simulink model "Controlled_PlanarRobot"  (R2021a)
settings: Solver=ode4  StartTime=0.0  StopTime=10  FixedStep=0.001  MaxStep=0.001  RelTol=1e-3
undefined symbols (not defined in the file): g, I1, I2, kr1, kr2, l1, lc1, lc2, m1, m2, th1, th1p1, th2, th2p1
settings Model: Creator=BODENBURG  LastModifiedBy=aka
settings DebuggingCC: AlgebraicLoopMsg=none  SFMachineParentedDataDiag=warning
settings SFSimCC: CustomCodeUndefinedFunction=UseInterfaceOnly

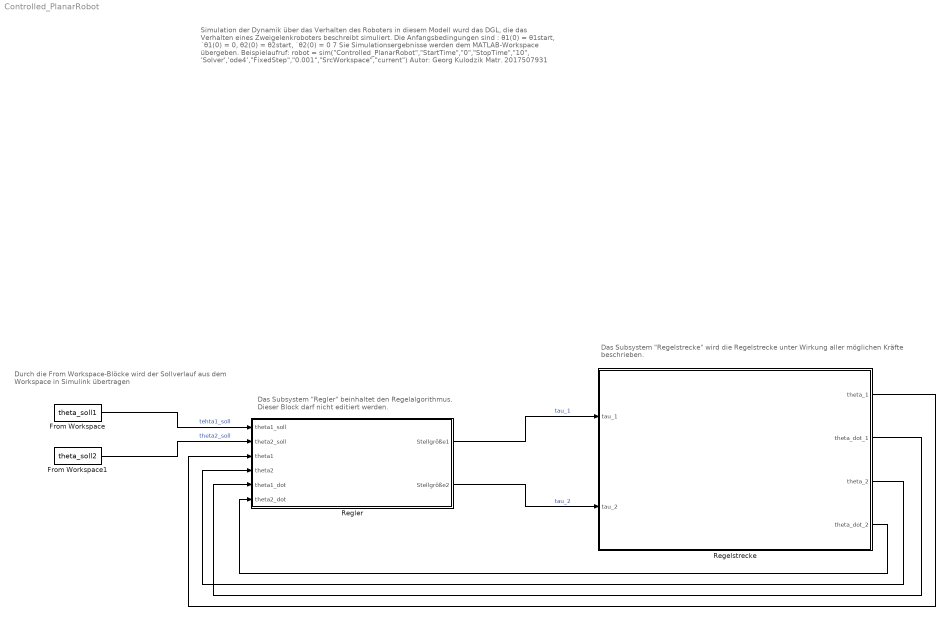
== system Controlled_PlanarRobot ==
  note: Durch die From Workspace-Blöcke wird der Sollverlauf aus dem Workspace in Simulink übertragen
  note: Das Subsystem "Regler" beinhaltet den Regelalgorithmus. Dieser Block darf nicht editiert werden.
  note: Simulation der Dynamik über das Verhalten des Roboters
      | in diesem Modell wurd das DGL,
      |
      | die das Verhalten eines Zweigelenkroboters beschreibt simuliert.
      | Die Anfangsbedingungen sind : θ1(0) = θ1start, ˙θ1(0) = 0, θ2(0) = θ2start, ˙θ2(0) = 0 7
      | Sie Simulationsergebnisse werden dem MATLAB-Workspace übergeben.
      |
      | Beispielaufruf: robot = sim("Controlled_PlanarRobot","StartTime","0","StopTime","10", 'Solver','ode4',"FixedStep","0.001","SrcWorkspace","current")
      |
      | Autor: Georg Kulodzik Matr. 2017507931
  note: Das Subsystem "Regelstrecke" wird die Regelstrecke unter Wirkung aller möglichen Kräfte beschrieben.
  From Workspace : FromWorkspace  VariableName=theta_soll1  OutputAfterFinalValue=Holding final value
  From Workspace1 : FromWorkspace  VariableName=theta_soll2  OutputAfterFinalValue=Holding final value
  Regelstrecke : Subsystem
  Regler : Subsystem
  wires:
  Regelstrecke/1(theta_1) -> Regler/3(theta1)
  Regelstrecke/3(theta_2) -> Regler/4(theta2)
  Regelstrecke/2(theta_dot_1) -> Regler/5(theta1_dot)
  Regelstrecke/4(theta_dot_2) -> Regler/6(theta2_dot)
  Regler/1(Stellgröße1) -> Regelstrecke/1(tau_1)  "tau_1"
  Regler/2(Stellgröße2) -> Regelstrecke/2(tau_2)  "tau_2"
  From Workspace/1 -> Regler/1(theta1_soll)  "tehta1_soll"
  From Workspace1/1 -> Regler/2(theta2_soll)  "theta2_soll"

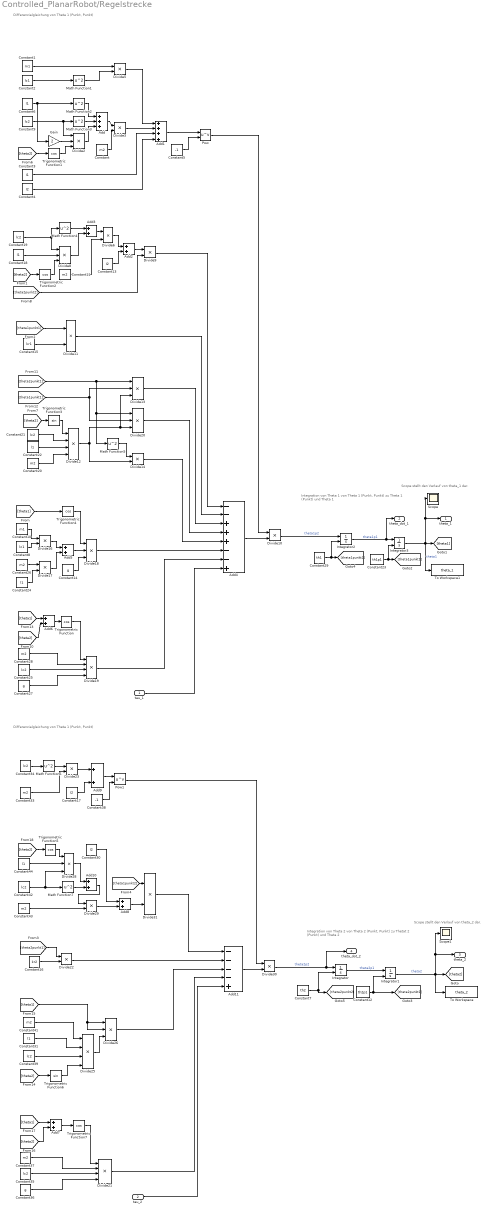
== system Controlled_PlanarRobot/Regelstrecke ==
  note: Integration von Theta 1 von Theta 1 (Punkt, Punkt)
      | zu Theta 1 (Punkt) und Theta 1
  note: Integration von Theta 2 von Theta 2 (Punkt, Punkt)
      | zu Thetat 2 (Punkt) und Theta 2
  note: Scope stellt den Verlauf von theta_1 dar.
  note: Scope stellt den Verlauf von theta_2 dar.
  note: Differenzialgleichung von Theta 1 (Punkt, Punkt)
  note: Differenzialgleichung von Theta 1 (Punkt, Punkt)
  tau_1 : Inport
  tau_2 : Inport  Port=2
  Add : Sum  Inputs=+++
  Add1 : Sum  Inputs=++++
  Add{2..3,5..10} (8 alike) : Sum
  Add11 : Sum  Inputs=----+
  Add4 : Sum  Inputs=--+++--+
  Constant{,11,20,26,28,33,37,41,43} (9 alike) : Constant  Value=m2
  Constant1 : Constant  Value=m1
  Constant10 : Constant  Value=m1
  Constant12 : Constant  Value=th2p1
  Constant{4,13,17,30} (4 alike) : Constant  Value=I2
  Constant14 : Constant  Value=g
  Constant15 : Constant  Value=kr1
  Constant16 : Constant  Value=kr2
  Constant{6,18,22,24,31,44} (6 alike) : Constant  Value=l1
  Constant{9,19,21,25,34..35,39,42} (8 alike) : Constant  Value=lc2
  Constant2 : Constant  Value=lc1
  Constant23 : Constant  Value=th1p1
  Constant27 : Constant  Value=g
  Constant29 : Constant  Value=th1
  Constant3 : Constant  Value=I1
  Constant36 : Constant  Value=g
  Constant38 : Constant  Value=-1
  Constant5 : Constant  Value=-1
  Constant7 : Constant  Value=th2
  Constant8 : Constant  Value=lc1
  Divide{3,5..6,9..11,14,16..17,22..23,29..31} (14 alike) : Product  Inputs=**
  Divide{12,19,21,25} (4 alike) : Product  Inputs=****
  Divide{2,8,13,18,20,26,28} (7 alike) : Product  Inputs=***
  Gain : Gain  Gain=2
  Integrator{,1..3} (4 alike) : Integrator  InitialConditionSource=external
  Math Function{1..7} (7 alike) : Math  Operator=square  SaturateOnIntegerOverflow=on
  Pow : Math  Operator=pow  SignedPower=on  RndMeth=Zero  SaturateOnIntegerOverflow=on
  Pow1 : Math  Operator=pow  SignedPower=on  RndMeth=Zero  SaturateOnIntegerOverflow=on
  Scope : Scope
  Scope1 : Scope
  To Workspace : ToWorkspace  VariableName=theta_2  SaveFormat=Timeseries  SampleTime=-1
  To Workspace1 : ToWorkspace  VariableName=theta_1  SaveFormat=Timeseries  SampleTime=-1
  Trigonometric Function{,1..2,4..5,7} (6 alike) : Trigonometry  Operator=cos
  Trigonometric Function3 : Trigonometry
  Trigonometric Function6 : Trigonometry
  theta_1 : Outport
  theta_dot_1 : Outport  Port=2
  theta_2 : Outport  Port=3
  theta_dot_2 : Outport  Port=4
  wires:
  Constant6/1 -> Math Function2/1, Gain/1
  Constant9/1 -> Math Function3/1, Divide2/1
  Trigonometric Function1/1 -> Divide2/3
  [theta2] -> Trigonometric Function1/1
  Divide2/1 -> Add/3
  Gain/1 -> Divide2/2
  Add/1 -> Divide3/1
  Constant/1 -> Divide3/2
  Constant1/1 -> Divide5/1
  Divide5/1 -> Add1/1
  Divide3/1 -> Add1/2
  Constant3/1 -> Add1/3
  Constant4/1 -> Add1/4
  Add1/1 -> Pow/1
  Constant5/1 -> Pow/2
  Divide6/1 -> Add2/1
  Constant13/1 -> Add2/2
  Constant11/1 -> Divide6/2
  Add3/1 -> Divide6/1
  Constant19/1 -> Math Function4/1, Divide8/1
  Divide8/1 -> Add3/2
  [theta2] -> Trigonometric Function2/1
  Trigonometric Function2/1 -> Divide8/3
  Constant18/1 -> Divide8/2
  [theta2punkt2] -> Divide9/2
  Pow/1 -> Divide10/1
  Add4/1 -> Divide10/2
  Add2/1 -> Divide9/1
  Constant15/1 -> Divide11/2
  [theta1punkt1] -> Divide11/1
  Constant20/1 -> Divide12/4
  Constant22/1 -> Divide12/3
  Constant21/1 -> Divide12/2
  [theta2] -> Trigonometric Function3/1
  Trigonometric Function3/1 -> Divide12/1
  Divide12/1 -> Divide14/2, Divide13/3, Divide20/3
  [theta2punkt1] -> Divide13/1, Math Function5/1, Divide20/1
  Constant10/1 -> Divide16/1
  Constant8/1 -> Divide16/2
  Constant26/1 -> Divide17/1
  Constant24/1 -> Divide17/2
  Divide16/1 -> Add5/1
  Divide17/1 -> Add5/2
  Add5/1 -> Divide18/2
  Trigonometric Function4/1 -> Divide18/1
  [theta1] -> Trigonometric Function4/1
  Constant14/1 -> Divide18/3
  Constant27/1 -> Divide19/4
  Constant25/1 -> Divide19/3
  Constant28/1 -> Divide19/2
  Trigonometric Function/1 -> Divide19/1
  [theta1] -> Add6/1
  [theta2] -> Add6/2
  Add6/1 -> Trigonometric Function/1
  Divide9/1 -> Add4/1
  Divide11/1 -> Add4/2
  Divide13/1 -> Add4/3
  [theta1punkt1] -> Divide13/2, Divide20/2
  Divide20/1 -> Add4/4
  Divide14/1 -> Add4/5
  Divide18/1 -> Add4/6
  tau_1/1 -> Add4/8
  Trigonometric Function7/1 -> Divide21/1
  Constant35/1 -> Divide21/3
  [theta1] -> Add7/1
  Add7/1 -> Trigonometric Function7/1
  Constant37/1 -> Divide21/2
  Constant36/1 -> Divide21/4
  [theta2] -> Add7/2
  Divide19/1 -> Add4/7
  [theta2punkt1] -> Divide22/1
  Constant33/1 -> Divide23/2
  Divide23/1 -> Add9/1
  Constant17/1 -> Add9/2
  Add9/1 -> Pow1/1
  Constant38/1 -> Pow1/2
  Constant41/1 -> Divide25/1
  Constant31/1 -> Divide25/2
  Constant39/1 -> Divide25/3
  [theta2] -> Trigonometric Function6/1
  Trigonometric Function6/1 -> Divide25/4
  Divide25/1 -> Divide26/3
  [theta1] -> Divide26/1, Divide26/2
  Constant16/1 -> Divide22/2
  Constant42/1 -> Divide28/3, Math Function7/1
  Divide28/1 -> Add10/1
  Constant44/1 -> Divide28/2
  Add10/1 -> Divide29/1
  Constant43/1 -> Divide29/2
  Divide22/1 -> Add11/2
  Divide26/1 -> Add11/3
  Divide21/1 -> Add11/4
  tau_2/1 -> Add11/5
  Pow1/1 -> Divide30/1
  Add11/1 -> Divide30/2
  Divide30/1 -> theta_dot_2/1, Integrator/1  "theta2p2"
  Integrator/1 -> Integrator1/1  "theta2p1"
  Constant7/1 -> Integrator/2, [theta2punkt2]
  Constant12/1 -> Integrator1/2, [theta2punkt1]
  Constant23/1 -> Integrator3/2, [theta1punkt1]
  Integrator2/1 -> theta_dot_1/1, Integrator3/1  "theta1p1"
  Constant29/1 -> [theta1punkt2], Integrator2/2
  Divide10/1 -> Integrator2/1  "theta1p2"
  Integrator3/1 -> Scope/1, theta_1/1, To Workspace1/1, [theta1]  "theta1"
  Integrator1/1 -> To Workspace/1, Scope1/1, theta_2/1, [theta2]  "theta2"
  Divide29/1 -> Add8/2
  Constant30/1 -> Add8/1
  Divide31/1 -> Add11/1
  Add8/1 -> Divide31/2
  [theta1punkt2] -> Divide31/1
  [theta2] -> Trigonometric Function5/1
  Trigonometric Function5/1 -> Divide28/1
  Math Function1/1 -> Divide5/2
  Constant2/1 -> Math Function1/1
  Math Function2/1 -> Add/1
  Math Function3/1 -> Add/2
  Math Function4/1 -> Add3/1
  Math Function5/1 -> Divide14/1
  Constant34/1 -> Math Function6/1
  Math Function6/1 -> Divide23/1
  Math Function7/1 -> Add10/2

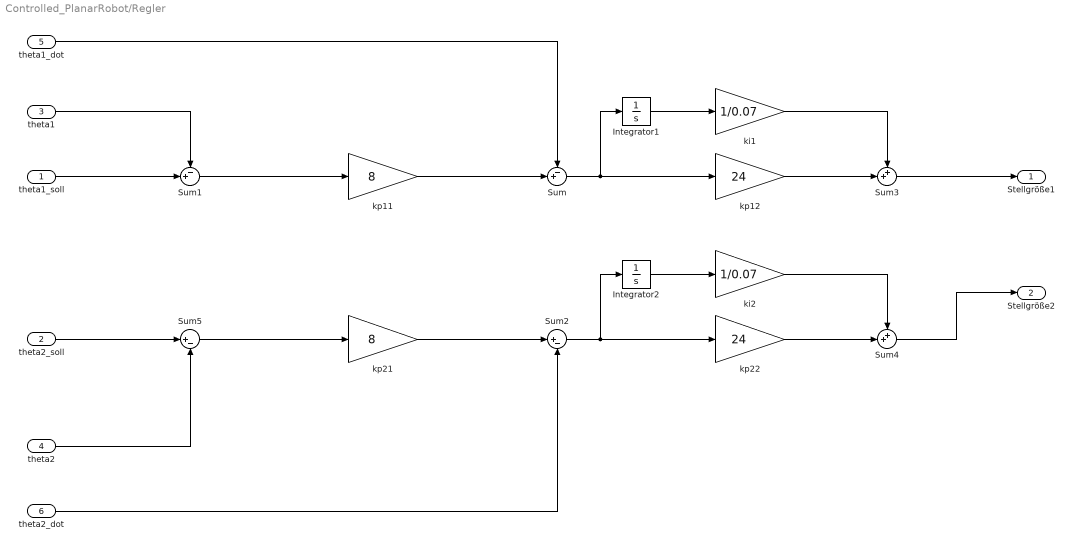
== system Controlled_PlanarRobot/Regler ==
  theta1_soll : Inport
  theta2_soll : Inport  Port=2
  theta1 : Inport  Port=3
  theta2 : Inport  Port=4
  theta1_dot : Inport  Port=5
  theta2_dot : Inport  Port=6
  Integrator1 : Integrator
  Integrator2 : Integrator
  Sum : Sum  Inputs=-+|
  Sum1 : Sum  Inputs=-+|
  Sum2 : Sum  Inputs=|+-
  Sum3 : Sum  Inputs=++|
  Sum4 : Sum  Inputs=++|
  Sum5 : Sum  Inputs=|+-
  ki1 : Gain  Gain=1/0.07
  ki2 : Gain  Gain=1/0.07
  kp11 : Gain  Gain=8
  kp12 : Gain  Gain=24
  kp21 : Gain  Gain=8
  kp22 : Gain  Gain=24
  Stellgröße1 : Outport
  Stellgröße2 : Outport  Port=2
  wires:
  Sum/1 -> kp12/1, Integrator1/1
  kp22/1 -> Sum4/2
  ki2/1 -> Sum4/1
  Integrator1/1 -> ki1/1
  kp11/1 -> Sum/2
  ki1/1 -> Sum3/1
  Sum5/1 -> kp21/1
  Integrator2/1 -> ki2/1
  theta2_dot/1 -> Sum2/2
  Sum2/1 -> kp22/1, Integrator2/1
  Sum1/1 -> kp11/1
  kp21/1 -> Sum2/1
  kp12/1 -> Sum3/2
  Sum4/1 -> Stellgröße2/1
  Sum3/1 -> Stellgröße1/1
  theta2_soll/1 -> Sum5/1
  theta1/1 -> Sum1/1
  theta1_soll/1 -> Sum1/2
  theta2/1 -> Sum5/2
  theta1_dot/1 -> Sum/1
